simulink model "myPLL_SOGI_R2023"  (R2023a)
settings: Solver=VariableStepAuto  StartTime=0.0  StopTime=1  MaxStep=1e-5  RelTol=1e-3
libraries: spsSeriesRLCBranchLib x2, slpidlib x1, spspowerguiLib x1
settings Model: Creator=JD  LastModifiedBy=JD
settings DebuggingCC: UnconnectedInputMsg=warning  UnconnectedOutputMsg=warning  UnconnectedLineMsg=warning
settings ModelReferenceCC: EnableRefExpFcnMdlSchedulingChecks=on
settings RTWCC: DLArmComputeVersion=19.05

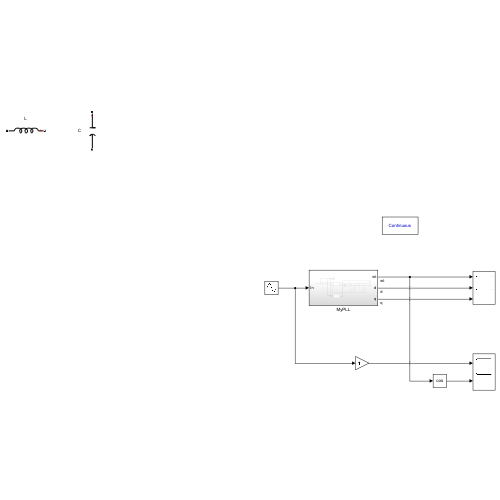
[thumbnail: Simulink's stored preview of the top-level diagram]
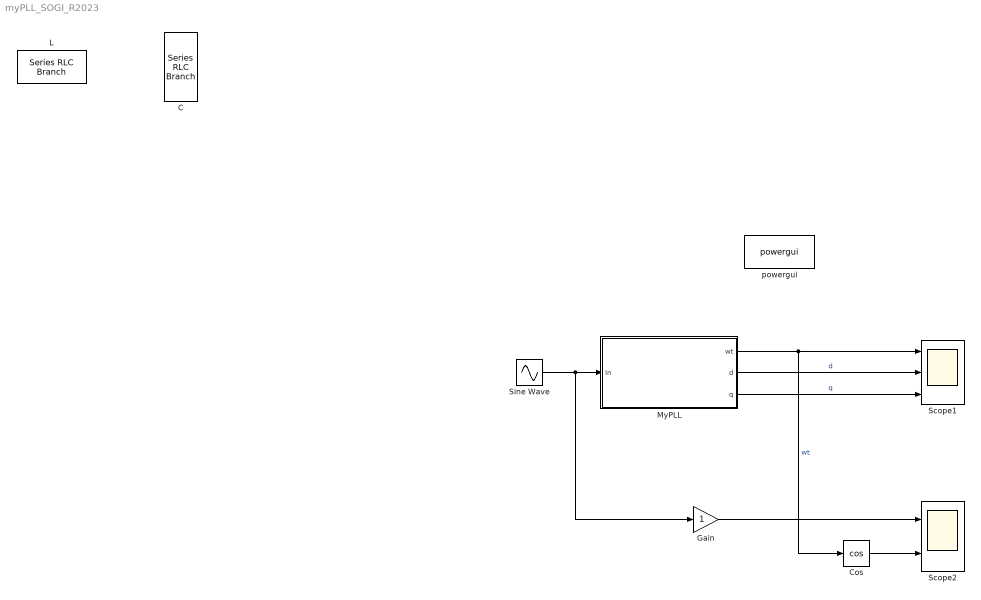
== system myPLL_SOGI_R2023 ==
  C : spsSeriesRLCBranchLib/Series RLC Branch  LConnTagsString=__new0  RConnTagsString=__new0  BranchType=C  Resistance=0.068  Inductance=1e-3  SetiL0=off  InitialCurrent=0  Capacitance=4e-3  Setx0=off  InitialVoltage=0  Measurements=Branch voltage
  Cos : Trigonometry  Operator=cos
  Gain : Gain
  L : spsSeriesRLCBranchLib/Series RLC Branch  LConnTagsString=__new0  RConnTagsString=__new0  BranchType=L  Resistance=0.068  Inductance=3e-3  SetiL0=off  InitialCurrent=0  Capacitance=1e-6  Setx0=off  InitialVoltage=0  Measurements=Branch current
  MyPLL : Subsystem
  Scope1 : Scope  NumInputPorts=3
  Scope2 : Scope  NumInputPorts=2
  Sine Wave : Sin  Amplitude=2  Frequency=50*2*pi  SampleTime=0
  powergui : spspowerguiLib/powergui  Priority=1  SimulationMode=Continuous  SampleTime=0.01/10000  frequency=60  Iterations=50  frequencyindice=50  Pbase=100e6  ErrMax=1e-4  UnitsV=kV  UnitsW=MW  buscounter=0  FunctionMessages=off  echomessages=off  EnableUseOfTLC=off  CurrentSourceSwitches=off  DisableSnubberDevices=off  DisableRonSwitches=off  DisableVfSwitches=off  DisplayEquations=off  AutomaticDiscreteSolvers=off  SolverType=Tustin/Backward Euler (TBE)  Interpol=off  ExternalGateDelay=off  methode=off  Ts=100  x0status=blocks  SPID=on  SwTol=0  HookPort=off  NonlinearTolerance=1e-4  nMaxIteration=100  ContinueOnMaxIteration=off  RestoreLinks=warning  ResistiveCurrentMeasurement=off  Frange=[0:2:500]  Ylog=off  Xlog=on  ShowGrid=off  save=off  variable=ZData  structure=0  ZoomFFT=off  StartTime=0.0  cycles=1  DisplayStyle=1  fundamental=60  FreqAxis=off  MaxFrequency=1000  frequencyindicesteady=1  RmsSteady=1  display=off
  wires:
  Sine Wave/1 -> Gain/1, MyPLL/1(In)
  MyPLL/1(wt) -> Scope1/1, Cos/1  "wt"
  MyPLL/2(d) -> Scope1/2  "d"
  MyPLL/3(q) -> Scope1/3  "q"
  Cos/1 -> Scope2/2
  Gain/1 -> Scope2/1

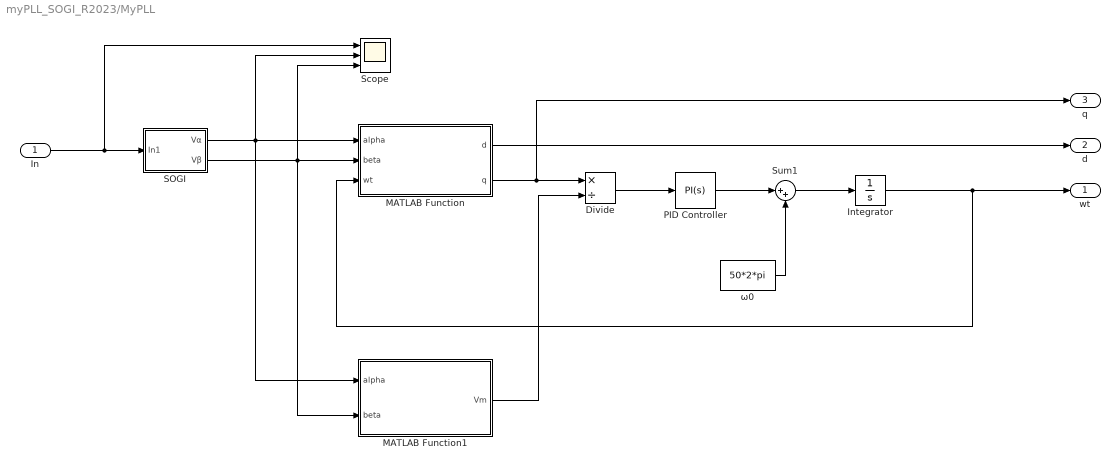
== system myPLL_SOGI_R2023/MyPLL ==
  In : Inport
  Divide : Product  Inputs=*/
  Integrator : Integrator  WrapState=on  WrappedStateUpperValue=2*pi  WrappedStateLowerValue=0
  MATLAB Function : MATLAB Function  TreatAsAtomicUnit=on
  MATLAB Function1 : MATLAB Function  TreatAsAtomicUnit=on
  PID Controller : slpidlib/PID Controller  Controller=PI  Form=Parallel  TimeDomain=Continuous-time  UseExternalTs=off  SampleTime=-1  IntegratorMethod=Forward Euler  FilterMethod=Forward Euler  ControllerParametersSource=internal  P=180  I=3200  UseKiTs=off  D=0  N=100  UseFilter=on  TunerSelectOption=Transfer Function Based (PID Tuner App)  InitialConditionSource=internal  InitialConditionForIntegrator=0  InitialConditionForFilter=0  DifferentiatorICPrevScaledInput=0  ExternalReset=none  TrackingMode=off  Kt=1  LimitOutput=off  SatLimitsSource=internal  UpperSaturationLimit=inf  LowerSaturationLimit=-inf  LinearizeAsGain=on  AntiWindupMode=none  Kb=1  LimitIntegrator=off  UpperIntegratorSaturationLimit=inf  LowerIntegratorSaturationLimit=-inf  POutMin=[]  POutMax=[]  IOutMin=[]  IOutMax=[]  DOutMin=[]  DOutMax=[]  NOutMin=[]  NOutMax=[]  SumOutMin=[]  SumOutMax=[]  SaturationOutMin=[]  SaturationOutMax=[]  PParamMin=[]  PParamMax=[]  IParamMin=[]  IParamMax=[]  DParamMin=[]  DParamMax=[]  NParamMin=[]  NParamMax=[]  KbParamMin=[]  KbParamMax=[]  KtParamMin=[]  KtParamMax=[]  KbOutMin=[]  KbOutMax=[]  KtOutMin=[]  KtOutMax=[]  IntegratorOutMin=[]  IntegratorOutMax=[]  FilterOutMin=[]  FilterOutMax=[]  SumI1OutMin=[]  SumI1OutMax=[]  SumI2OutMin=[]  SumI2OutMax=[]  SumI3OutMin=[]  SumI3OutMax=[]  SumI4OutMin=[]  SumI4OutMax=[]  SumDOutMin=[]  SumDOutMax=[]  DifferentiatorOutMin=[]  DifferentiatorOutMax=[]  FilterDiffOutCoefMin=[]  FilterDiffOutCoefMax=[]  ReciprocalOutMin=[]  ReciprocalOutMax=[]  SumDenOutMin=[]  SumDenOutMax=[]  SumNumOutMin=[]  SumNumOutMax=[]  DivideOutMin=[]  DivideOutMax=[]  UdiffTsProdOutMin=[]  UdiffTsProdOutMax=[]  NTsProdOutMin=[]  NTsProdOutMax=[]  UintegralTsProdOutMin=[]  UintegralTsProdOutMax=[]  UngainTsProdOutMin=[]  UngainTsProdOutMax=[]  ClampingZeroOutDataTypeStr=Inherit: Inherit via back propagation  ClampingZeroOutMin=[]  ClampingZeroOutMax=[]  FilterDenConstantOutDataTypeStr=Inherit: Inherit via back propagation  FilterDenConstantOutMin=[]  FilterDenConstantOutMax=[]  PCopyOutDataTypeStr=Inherit: Inherit via back propagation  PCopyOutMin=[]  PCopyOutMax=[]  NCopyOutDataTypeStr=Inherit: Inherit via back propagation  NCopyOutMin=[]  NCopyOutMax=[]  IntegratorContinuousStateAttributes=''  IntegratorStateMustResolveToSignalObject=off  IntegratorRTWStateStorageClass=Auto  FilterContinuousStateAttributes=''  FilterStateMustResolveToSignalObject=off  FilterRTWStateStorageClass=Auto  ParallelPVariant=InternalParameters  IdealPVariant=Disabled  IVariant=InternalParameters  DVariant=Disabled  IntegratorVariant=Continuous  SatVariant=Disabled  AWVariant=Passthrough  PCopyVariant=Disabled  TRVariant=Disabled  FdbkBlocksVariant=Forward  IdealPFdbkVariant=Disabled  SatFdbkVariant=Disabled  DerivativeFilterVariant=Disabled  NVariant=Disabled  NCopyVariant=Disabled_SignalSpec  FilterICVariant=Disabled  IntegratorICVariant=InternalICs  ExternalResetVariant=Disabled  TRSumVariant=Passthrough  SumFdbkVariant=Disabled  SumVariant=Sum_PI  TsampFilterVariant=InternalTs  TsampNgainVariant=Passthrough  TsampIntegralVariant=Disabled_SignalSpec  ExternalSaturationOutDataTypeStr=Inherit: Same as second input
  SOGI : Subsystem
  Scope : Scope  NumInputPorts=3
  Sum1 : Sum  Inputs=|++
  ω0 : Constant  Value=50*2*pi
  wt : Outport
  d : Outport  Port=2
  q : Outport  Port=3
  wires:
  SOGI/1(Vα) -> Scope/2, MATLAB Function/1(alpha), MATLAB Function1/1(alpha)
  In/1 -> Scope/1, SOGI/1(In1)
  ω0/1 -> Sum1/2
  SOGI/2(Vβ) -> Scope/3, MATLAB Function/2(beta), MATLAB Function1/2(beta)
  PID Controller/1 -> Sum1/1
  Integrator/1 -> MATLAB Function/3(wt), wt/1
  MATLAB Function/2(q) -> q/1, Divide/1
  Sum1/1 -> Integrator/1
  Divide/1 -> PID Controller/1
  MATLAB Function1/1(Vm) -> Divide/2
  MATLAB Function/1(d) -> d/1

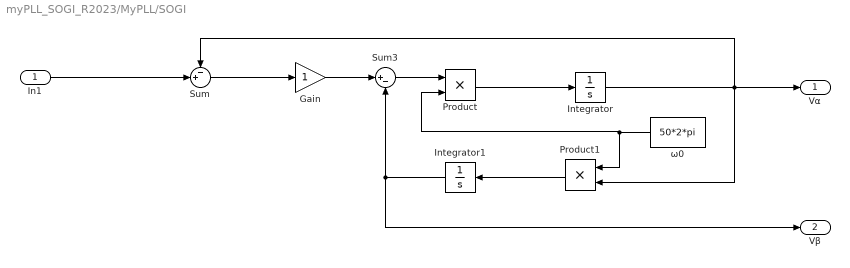
== system myPLL_SOGI_R2023/MyPLL/SOGI ==
  In1 : Inport
  Gain : Gain
  Integrator : Integrator
  Integrator1 : Integrator
  Product : Product
  Product1 : Product
  Sum : Sum  Inputs=-+|
  Sum3 : Sum  Inputs=|+-
  ω0 : Constant  Value=50*2*pi
  Vα : Outport
  Vβ : Outport  Port=2
  wires:
  Integrator/1 -> Vα/1, Sum/1, Product1/2
  In1/1 -> Sum/2
  Integrator1/1 -> Vβ/1, Sum3/2
  Gain/1 -> Sum3/1
  Sum3/1 -> Product/1
  Product/1 -> Integrator/1
  Sum/1 -> Gain/1
  Product1/1 -> Integrator1/1
  ω0/1 -> Product1/1, Product/2

== matlab function myPLL_SOGI_R2023/MyPLL/MATLAB Function1 ==
  data: alpha input; Vm output; beta input
function Vm = getModulus(alpha, beta)

Vm = max(0.1, sqrt(alpha ^ 2 + beta ^ 2));

== matlab function myPLL_SOGI_R2023/MyPLL/MATLAB Function ==
  data: alpha input; d output; beta input; wt input; q output
function [d, q] = DQ_Transform(alpha, beta, wt)

d = alpha * cos(wt) + beta * sin(wt);
q = -alpha * sin(wt) + beta * cos(wt);
